simulink model "simple_motor_mdl"  (R2020b)
settings: Solver=VariableStepAuto  StartTime=0.0  StopTime=10.0  RelTol=1e-3
model mask{Kv=670, R=.04, io=3.9}
  mask prompts: Kv "Speed constant, Kv [RPM/V]:"; R "Resistance [ohm]:"; io "Idle current [A]:"
model workspace (MAT data in the model file):
  Kv = Simulink.Parameter
  Kv.Value = 670
  Kv.DataType = 'auto'
  Kv.Dimensions = [1 1]
  R = Simulink.Parameter
  R.Value = 0.04
  R.DataType = 'auto'
  R.Dimensions = [1 1]
  io = Simulink.Parameter
  io.Value = 3.9
  io.DataType = 'auto'
  io.Dimensions = [1 1]
settings Model: ParameterArgumentNames=Kv,R,io  OrderedModelArguments=off  Creator=brian  LastModifiedBy=brian

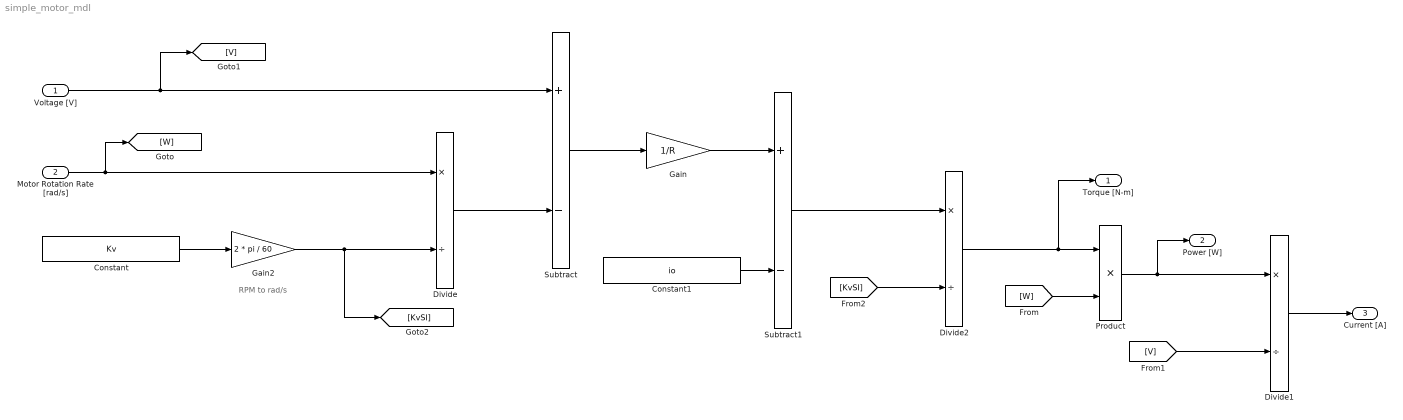
== system simple_motor_mdl ==
  note: RPM to rad/s
  Voltage [V] : Inport
  Motor Rotation Rate [rad/s] : Inport  Port=2
  Constant : Constant  Value=Kv
  Constant1 : Constant  Value=io
  Divide : Product  Inputs=*/
  Divide1 : Product  Inputs=*/
  Divide2 : Product  Inputs=*/
  Gain : Gain  Gain=1/R
  Gain2 : Gain  Gain=2 * pi / 60
  Product : Product
  Subtract : Sum  Inputs=+-
  Subtract1 : Sum  Inputs=+-
  Torque [N-m] : Outport
  Power [W] : Outport  Port=2
  Current [A] : Outport  Port=3
  wires:
  Motor Rotation Rate [rad/s]/1 -> [W], Divide/1
  Divide/1 -> Subtract/2
  Voltage [V]/1 -> [V], Subtract/1
  Subtract/1 -> Gain/1
  Gain/1 -> Subtract1/1
  Constant1/1 -> Subtract1/2
  Subtract1/1 -> Divide2/1
  Divide2/1 -> Product/1, Torque [N-m]/1
  [W] -> Product/2
  Product/1 -> Divide1/1, Power [W]/1
  [V] -> Divide1/2
  Divide1/1 -> Current [A]/1
  Constant/1 -> Gain2/1
  Gain2/1 -> [KvSI], Divide/2
  [KvSI] -> Divide2/2
